simulink model "pratica12S"  (R2021b)
settings: Solver=VariableStepAuto  StartTime=0.0  StopTime=24.00  RelTol=1e-3
values from neighbouring files (symbols this model uses):
  L = transpose(Lt)    [pratica12.m]
  R = 1.15    [pratica12.m]
  T0 = (2*pi)/ws    [pratica12.m]
undefined symbols (not defined in the file or in its folder): Cd, F, H
settings Model: Creator=carlo  LastModifiedBy=11800559

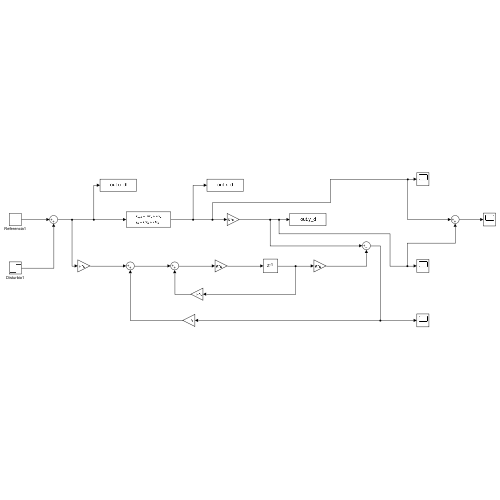
[thumbnail: Simulink's stored preview of the top-level diagram]
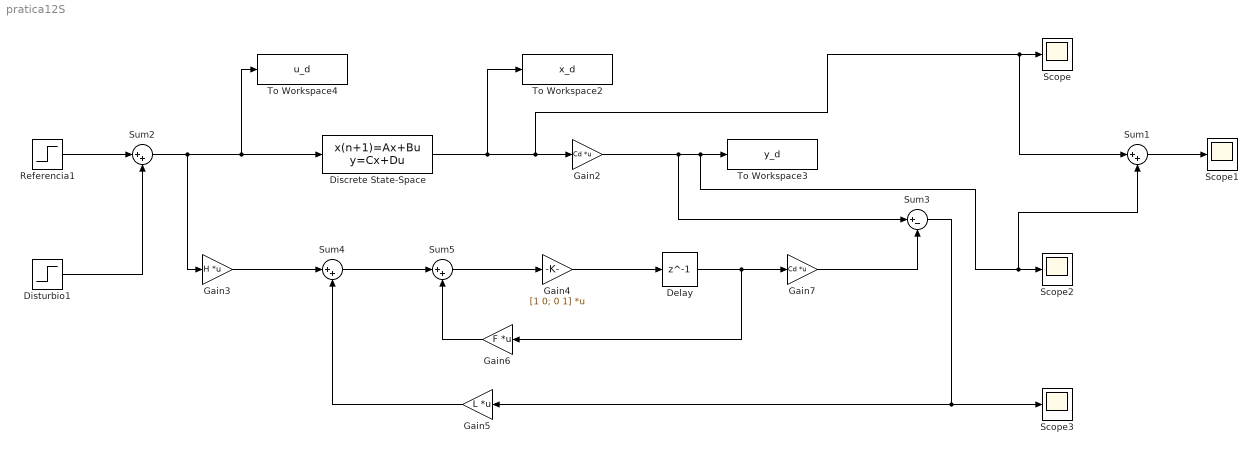
== system pratica12S ==
  Delay : Delay  DelayLength=1  InitialCondition=0
  Discrete State-Space : DiscreteStateSpace  A=F  B=H  C=[1 0; 0 1]  D=[0 ; 0]  SampleTime=T0
  Disturbio1 : Step  Time=0  After=R  SampleTime=0
  Gain2 : Gain  Gain=Cd  Multiplication=Matrix(K*u)
  Gain3 : Gain  Gain=H  Multiplication=Matrix(K*u)
  Gain4 : Gain  Gain=[1 0; 0 1]  Multiplication=Matrix(K*u)
  Gain5 : Gain  Gain=L  Multiplication=Matrix(K*u)
  Gain6 : Gain  Gain=F  Multiplication=Matrix(K*u)
  Gain7 : Gain  Gain=Cd  Multiplication=Matrix(K*u)
  Referencia1 : Step  Time=0  After=R  SampleTime=0
  Scope{,1..3} (4 alike) : Scope
  Sum{1..2,4..5} (4 alike) : Sum  Inputs=|++
  Sum3 : Sum  Inputs=|+-
  To Workspace2 : ToWorkspace  VariableName=x_d  SaveFormat=Timeseries  SampleTime=-1
  To Workspace3 : ToWorkspace  VariableName=y_d  SaveFormat=Timeseries  SampleTime=-1
  To Workspace4 : ToWorkspace  VariableName=u_d  SaveFormat=Timeseries  SampleTime=-1
  wires:
  Gain5/1 -> Sum4/2
  Sum5/1 -> Gain4/1
  Sum4/1 -> Sum5/1
  Gain6/1 -> Sum5/2
  Gain7/1 -> Sum3/2
  Sum3/1 -> Gain5/1, Scope3/1
  Sum2/1 -> Gain3/1, To Workspace4/1, Discrete State-Space/1
  Delay/1 -> Gain6/1, Gain7/1
  Gain3/1 -> Sum4/1
  Gain4/1 -> Delay/1
  Gain2/1 -> Sum1/2, Scope2/1, To Workspace3/1, Sum3/1
  Discrete State-Space/1 -> To Workspace2/1, Sum1/1, Scope/1, Gain2/1
  Referencia1/1 -> Sum2/1
  Disturbio1/1 -> Sum2/2
  Sum1/1 -> Scope1/1
